simulink model "Full_RC_2"  (Simulink 8.3)
settings: Solver=ode45  StartTime=0.0  StopTime=300000.0  RelTol=1e-3
settings Model: Creator=user  LastModifiedBy=user
settings DataIOCC: SignalLoggingSaveFormat=Dataset
settings DebuggingCC: UnderspecifiedInitializationDetection=Simplified  StateNameClashWarn=none
settings GRTTargetCC: CombineOutputUpdateFcns=on  GRTInterface=off

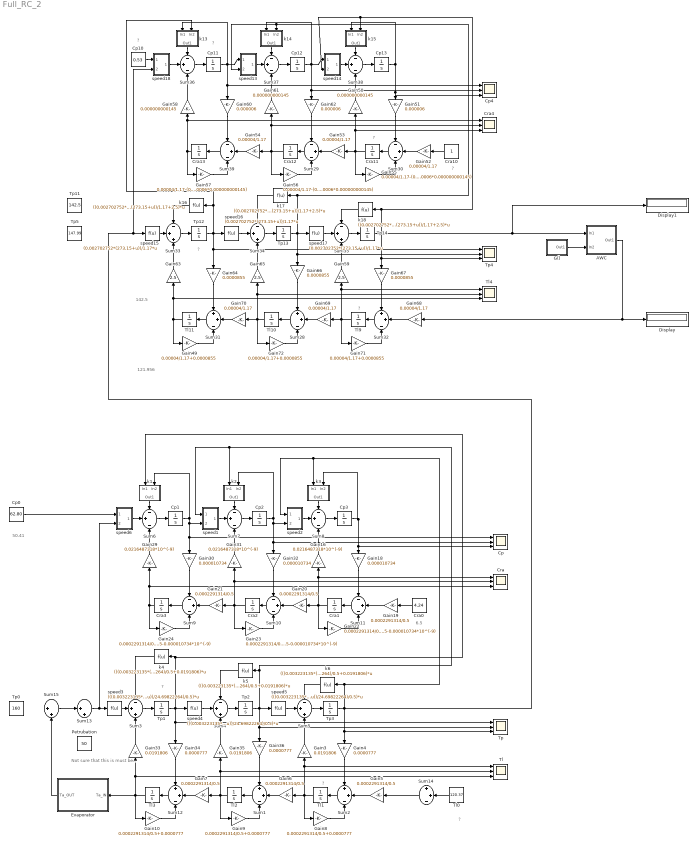
== system Full_RC_2 ==
  note: ?
  note: ?
  note: ?
  note: ?
  note: ?
  note: ?
  note: ?
  note: ?
  note: ?
  note: 50.41
  note: 6.5
  note: 142.5
  note: 121.956
  note: Not sure that
      | this is must be..
  AWC : Subsystem
  Cp : Scope  NumInputPorts=3
      settings: TimeRange=12  YMin=61.5~77~95.34999999999999  YMax=62.5~82~95.37000000000001  SaveName=Cp  DataFormat=Structure
  Cp0 : Constant  Value=62.80
  Cp1 : Integrator  InitialCondition=62.80
  Cp10 : Constant  Value=0.53
  Cp11 : Integrator  InitialCondition=0.665
  Cp12 : Integrator  InitialCondition=0.803
  Cp13 : Integrator  InitialCondition=0.986
  Cp2 : Integrator  InitialCondition=77.79
  Cp3 : Integrator  InitialCondition=96.56
  Cp4 : Scope  NumInputPorts=3
      settings: TimeRange=12  YMin=61.5~77~95.34999999999999  YMax=62.5~82~95.37000000000001  SaveName=Cp1  DataFormat=Structure
  Cra : Scope  NumInputPorts=3
      settings: YMin=4.17~2.4~0.84  YMax=4.28~2.5~1  SaveName=Cra
  Cra0 : Constant  Value=4.24
  Cra1 : Integrator  InitialCondition=4.24
  Cra10 : Constant
  Cra11 : Integrator  InitialCondition=0.827
  Cra12 : Integrator  InitialCondition=0.6862
  Cra13 : Integrator  InitialCondition=0.5696
  Cra2 : Integrator  InitialCondition=2.42
  Cra3 : Integrator  InitialCondition=0.95
  Cra4 : Scope  NumInputPorts=3
      settings: YMin=4.17~2.4~0.84  YMax=4.28~2.5~1  SaveName=Cra1
  Display : Display
  Display1 : Display
  Evaporator : Subsystem
  G() : Subsystem
  Gain10 : Gain  Gain=0.0002291314/0.5+0.0000777
  Gain16 : Gain  Gain=0.0216487318*10^(-9)
  Gain18 : Gain  Gain=0.000010734
  Gain{5..7,19..21} (6 alike) : Gain  Gain=0.0002291314/0.5
  Gain22 : Gain  Gain=0.0002291314/0.5-0.000010734*10^(-9)
  Gain23 : Gain  Gain=0.0002291314/0.5-0.000010734*10^(-9)
  Gain24 : Gain  Gain=0.0002291314/0.5-0.000010734*10^(-9)
  Gain29 : Gain  Gain=0.0216487318*10^(-9)
  Gain3 : Gain  Gain=0.0191806
  Gain30 : Gain  Gain=0.000010734
  Gain31 : Gain  Gain=0.0216487318*10^(-9)
  Gain32 : Gain  Gain=0.000010734
  Gain33 : Gain  Gain=0.0191806
  Gain34 : Gain  Gain=0.0000777
  Gain35 : Gain  Gain=0.0191806
  Gain36 : Gain  Gain=0.0000777
  Gain4 : Gain  Gain=0.0000777
  Gain49 : Gain  Gain=0.00004/1.17+0.0000855
  Gain50 : Gain  Gain=0.000000000145
  Gain51 : Gain  Gain=0.000006
  Gain{52..54,68..70} (6 alike) : Gain  Gain=0.00004/1.17
  Gain55 : Gain  Gain=0.00004/1.17-(0.000006*0.000000000145)
  Gain56 : Gain  Gain=0.00004/1.17-(0.000006*0.000000000145)
  Gain57 : Gain  Gain=0.00004/1.17-(0.000006*0.000000000145)
  Gain58 : Gain  Gain=0.000000000145
  Gain59 : Gain  Gain=2.5
  Gain60 : Gain  Gain=0.000006
  Gain61 : Gain  Gain=0.000000000145
  Gain62 : Gain  Gain=0.000006
  Gain63 : Gain  Gain=2.5
  Gain64 : Gain  Gain=0.0000855
  Gain65 : Gain  Gain=2.5
  Gain66 : Gain  Gain=0.0000855
  Gain67 : Gain  Gain=0.0000855
  Gain71 : Gain  Gain=0.00004/1.17+0.0000855
  Gain72 : Gain  Gain=0.00004/1.17+0.0000855
  Gain8 : Gain  Gain=0.0002291314/0.5+0.0000777
  Gain9 : Gain  Gain=0.0002291314/0.5+0.0000777
  Petrubation : Constant  Value=50
  Sum{1..2,12,14,28,31..32} (7 alike) : Sum  Inputs=++-
  Sum{6..11,29..30,36..39} (12 alike) : Sum  Inputs=-+-
  Sum13 : Sum  Inputs=|++
  Sum15 : Sum  Inputs=|++
  Sum{3..5,33..35} (6 alike) : Sum  Inputs=-++
  Tl : Scope  NumInputPorts=3
      settings: YMin=13~10~8.800000000000001  YMax=15.2~21~10.55  SaveName=Tl
  Tl0 : Constant  Value=120.37
  Tl1 : Integrator  InitialCondition=120.37
  Tl10 : Integrator  InitialCondition=86.23
  Tl11 : Integrator  InitialCondition=111.75
  Tl2 : Integrator  InitialCondition=124.37
  Tl3 : Integrator  InitialCondition=128.38
  Tl4 : Scope  NumInputPorts=3
      settings: YMin=13~10~8.800000000000001  YMax=15.2~21~10.55  SaveName=Tl1
  Tl9 : Integrator  InitialCondition=58.28
  Tp : Scope  NumInputPorts=3
      settings: TimeRange=12  YMin=155.5~145~146  YMax=158.5~152~154.5  SaveName=Tp
  Tp0 : Constant  Value=160
  Tp1 : Integrator  InitialCondition=160
  Tp11 : Constant  Value=142.5
  Tp12 : Integrator  InitialCondition=121.956
  Tp13 : Integrator  InitialCondition=97.4
  Tp14 : Integrator  InitialCondition=69.6  IgnoreLimit=on
  Tp2 : Integrator  InitialCondition=157.34
  Tp3 : Integrator  InitialCondition=153.75  IgnoreLimit=on
  Tp4 : Scope  NumInputPorts=3
      settings: TimeRange=12  YMin=123.005~98.3982~69.9473  YMax=135.953~108.756~77.3101  SaveName=Tp1
  Tp5 : Constant  Value=147.99
  k1 : Subsystem
  k13 : Subsystem
  k14 : Subsystem
  k15 : Subsystem
  k16 : Fcn  Expr=((0.002702752*(273.15+u))/1.17+2.5)*u
  k17 : Fcn  Expr=((0.002702752*(273.15+u))/1.17+2.5)*u
  k18 : Fcn  Expr=((0.002702752*(273.15+u))/1.17+2.5)*u
  k2 : Subsystem
  k3 : Subsystem
  k4 : Fcn  Expr=(((0.003223135*(273+u))/24.69822264)/0.5+0.0191806)*u
  k5 : Fcn  Expr=(((0.003223135*(273+u))/24.69822264)/0.5+0.0191806)*u
  k6 : Fcn  Expr=(((0.003223135*(273+u))/24.69822264)/0.5+0.0191806)*u
  speed1 : Subsystem
  speed13 : Subsystem
  speed14 : Subsystem
  speed15 : Fcn  Expr=(0.002702752*(273.15+u))/1.17*u
  speed16 : Fcn  Expr=(0.002702752*(273.15+u))/1.17*u
  speed17 : Fcn  Expr=(0.002702752*(273.15+u))/1.17*u
  speed18 : Subsystem
  speed2 : Subsystem
  speed3 : Fcn  Expr=(((0.003223135*(273+u))/24.69822264)/0.5)*u
  speed4 : Fcn  Expr=(((0.003223135*(273+u))/24.69822264)/0.5)*u
  speed5 : Fcn  Expr=(((0.003223135*(273+u))/24.69822264)/0.5)*u
  speed6 : Subsystem
  wires:
  Sum6/1 -> Cp1/1
  speed1/1(Out1) -> Sum7/2
  Sum7/1 -> Cp2/1
  speed2/1(Out1) -> Sum8/2
  Sum8/1 -> Cp3/1
  Cp1/1 -> speed1/2(In2), Gain30/1, Cp/1, k1/2(In2)
  Cp2/1 -> speed2/2(In2), Gain32/1, Cp/2, k2/2(In2)
  Gain29/1 -> Sum6/3
  Cp3/1 -> k3/2(In2), Gain18/1, Cp/3
  Gain31/1 -> Sum7/3
  Gain16/1 -> Sum8/3
  Gain30/1 -> Sum9/1
  Gain32/1 -> Sum10/1
  Gain18/1 -> Sum11/1
  Gain19/1 -> Sum11/2
  Sum11/1 -> Cra1/1
  Cra1/1 -> Gain22/1, Gain20/1, Gain16/1, Cra/1
  Gain20/1 -> Sum10/2
  Sum10/1 -> Cra2/1
  Cra2/1 -> Gain23/1, Gain21/1, Gain31/1, Cra/2
  Gain21/1 -> Sum9/2
  Sum9/1 -> Cra3/1
  Cra3/1 -> Gain24/1, Gain29/1, Cra/3
  Gain22/1 -> Sum11/3
  Gain23/1 -> Sum10/3
  Gain24/1 -> Sum9/3
  speed3/1 -> Sum3/2
  k4/1 -> Sum3/1
  Sum3/1 -> Tp1/1
  speed4/1 -> Sum4/2
  k5/1 -> Sum4/1
  Sum4/1 -> Tp2/1
  speed5/1 -> Sum5/2
  k6/1 -> Sum5/1
  Sum5/1 -> Tp3/1
  Gain33/1 -> Sum3/3
  Tp3/1 -> Gain4/1, Tp/3, speed18/2(In2), speed15/1, k6/1, k3/1(In1), speed2/1(In1)
  Gain35/1 -> Sum4/3
  Gain3/1 -> Sum5/3
  Gain34/1 -> Sum12/1
  Gain36/1 -> Sum1/1
  Gain4/1 -> Sum2/1
  Gain5/1 -> Sum2/2
  Sum2/1 -> Tl1/1
  Tl1/1 -> Gain8/1, Gain6/1, Gain3/1, Tl/1
  Gain6/1 -> Sum1/2
  Sum1/1 -> Tl2/1
  Tl2/1 -> Gain9/1, Gain7/1, Gain35/1, Tl/2
  Gain7/1 -> Sum12/2
  Sum12/1 -> Tl3/1
  Tl3/1 -> Evaporator/1(Ta_IN), Gain10/1, Gain33/1, Tl/3
  Gain8/1 -> Sum2/3
  Gain9/1 -> Sum1/3
  Gain10/1 -> Sum12/3
  speed6/1(Out1) -> Sum6/2
  Cp0/1 -> speed6/1(In1)
  k1/1(Out1) -> Sum6/1
  k2/1(Out1) -> Sum7/1
  k3/1(Out1) -> Sum8/1
  Cra0/1 -> Gain19/1
  Sum13/1 -> speed6/2(In2), speed3/1
  G()/1(Out1) -> AWC/2(In2)
  Sum14/1 -> Gain5/1
  Sum15/1 -> Sum13/1
  Tl0/1 -> Sum14/2
  Tp2/1 -> Gain36/1, Tp/2, k5/1, speed1/1(In1), k2/1(In1), speed5/1
  Tp1/1 -> Gain34/1, Tp/1, k4/1, k1/1(In1), speed4/1
  Evaporator/1(Ta_OUT) -> Sum15/2
  Sum36/1 -> Cp11/1
  speed13/1(Out1) -> Sum37/2
  Sum37/1 -> Cp12/1
  speed14/1(Out1) -> Sum38/2
  Sum38/1 -> Cp13/1
  Cp11/1 -> Cp4/1, Gain60/1, speed13/1(In1), k13/1(In1)
  Cp12/1 -> Cp4/2, Gain62/1, speed14/1(In1), k14/1(In1)
  Gain58/1 -> Sum36/3
  Cp13/1 -> Cp4/3, Gain51/1, k15/1(In1)
  Gain61/1 -> Sum37/3
  Gain50/1 -> Sum38/3
  Gain60/1 -> Sum39/1
  Gain62/1 -> Sum29/1
  Gain51/1 -> Sum30/1
  Gain52/1 -> Sum30/2
  Sum30/1 -> Cra11/1
  Cra11/1 -> Gain55/1, Gain53/1, Cra4/3, Gain50/1
  Gain53/1 -> Sum29/2
  Sum29/1 -> Cra12/1
  Cra12/1 -> Gain56/1, Gain54/1, Cra4/2, Gain61/1
  Gain54/1 -> Sum39/2
  Sum39/1 -> Cra13/1
  Cra13/1 -> Gain57/1, Cra4/1, Gain58/1
  Gain55/1 -> Sum30/3
  Gain56/1 -> Sum29/3
  Gain57/1 -> Sum39/3
  speed15/1 -> Sum33/2
  k16/1 -> Sum33/1
  Sum33/1 -> Tp12/1
  speed16/1 -> Sum34/2
  k17/1 -> Sum34/1
  Sum34/1 -> Tp13/1
  speed17/1 -> Sum35/2
  k18/1 -> Sum35/1
  Sum35/1 -> Tp14/1
  Tp12/1 -> Gain64/1, Tp4/1, k16/1, k13/2(In2), speed16/1
  Tp13/1 -> Gain66/1, Tp4/2, k17/1, speed13/2(In2), k14/2(In2), speed17/1
  Gain63/1 -> Sum33/3
  Gain65/1 -> Sum34/3
  Gain59/1 -> Sum35/3
  Gain64/1 -> Sum31/1
  Gain66/1 -> Sum28/1
  Gain67/1 -> Sum32/1
  Gain68/1 -> Sum32/2
  Sum32/1 -> Tl9/1
  Tl9/1 -> Gain71/1, Gain69/1, Tl4/1, Gain59/1
  Gain69/1 -> Sum28/2
  Sum28/1 -> Tl10/1
  Tl10/1 -> Gain72/1, Gain70/1, Tl4/2, Gain65/1
  Gain70/1 -> Sum31/2
  Sum31/1 -> Tl11/1
  Tl11/1 -> Gain49/1, Gain63/1, Tl4/3
  Gain71/1 -> Sum32/3
  Gain72/1 -> Sum28/3
  Gain49/1 -> Sum31/3
  speed18/1(Out1) -> Sum36/2
  Cp10/1 -> speed18/1(In1)
  k13/1(Out1) -> Sum36/1
  k14/1(Out1) -> Sum37/1
  k15/1(Out1) -> Sum38/1
  Cra10/1 -> Gain52/1
  Tp14/1 -> AWC/1(In1), Display1/1, Gain67/1, Tp4/3, k18/1, k15/2(In2), speed14/2(In2)
  AWC/1(Out1) -> Display/1, Gain68/1

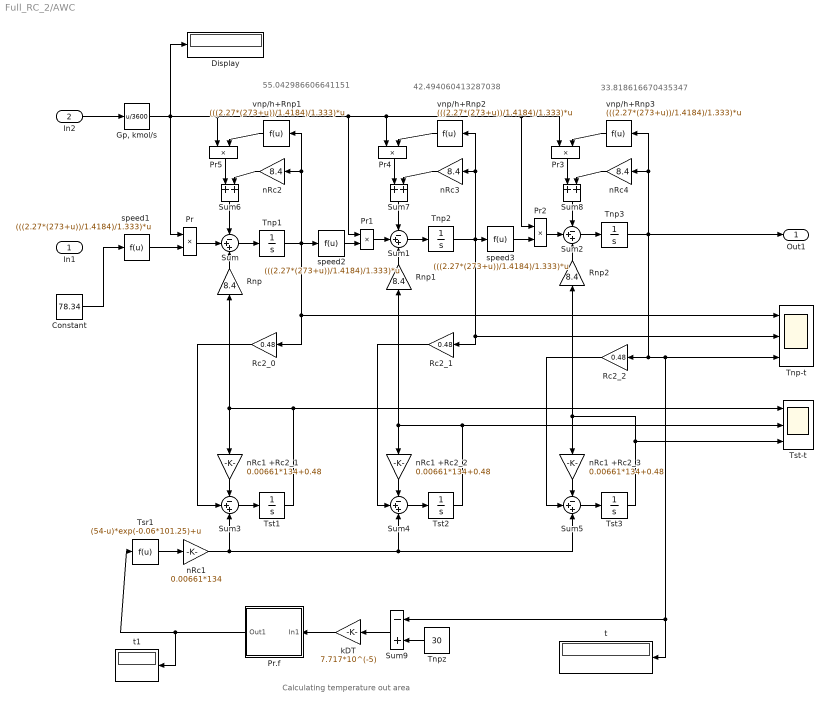
== system Full_RC_2/AWC ==
  note: 33.818616670435347
  note: 42.494060413287038
  note: 55.042986606641151
  note: Calculating temperature out area
  In1 : Inport
  In2 : Inport  Port=2
  Constant : Constant  Value=78.34
  Display : Display
  "Gp, kmol/s" : Fcn  Expr=u/3600
  Pr{,1..5} (6 alike) : Product  RndMeth=Zero
  Pr.f : Subsystem
  Rc2_0 : Gain  Gain=0.48
  Rc2_1 : Gain  Gain=0.48
  Rc2_2 : Gain  Gain=0.48
  Rnp : Gain  Gain=8.4
  Rnp1 : Gain  Gain=8.4
  Rnp2 : Gain  Gain=8.4
  Sum{,1..5} (6 alike) : Sum  Inputs=-++
  Sum6 : Sum
  Sum7 : Sum
  Sum8 : Sum
  Sum9 : Sum  Inputs=-+
  Tnp-t : Scope  NumInputPorts=3
      settings: YMin=52.458~37.745~29.975  YMax=52.466~37.7725~30.025  SaveName=ScopeData8
  Tnp1 : Integrator  InitialCondition=55.042986606641151
  Tnp2 : Integrator  InitialCondition=42.494060413287038
  Tnp3 : Integrator  InitialCondition=33.818616670435347
  Tnpz : Constant  Value=30
  Tsr1 : Fcn  Expr=(54-u)*exp(-0.06*101.25)+u
  Tst-t : Scope  NumInputPorts=3
      settings: YMin=320.767~573.618~826.668  YMax=354.532~633.998~913.686  SaveName=ScopeData9
  Tst1 : Integrator  InitialCondition=30.749212884999000
  Tst2 : Integrator  InitialCondition=26.338794670104530
  Tst3 : Integrator  InitialCondition=23.289742144317184
  kDT : Gain  Gain=7.717*10^(-5)
  nRc1 : Gain  Gain=0.00661*134
  nRc1 +Rc2_1 : Gain  Gain=0.00661*134+0.48
  nRc1 +Rc2_2 : Gain  Gain=0.00661*134+0.48
  nRc1 +Rc2_3 : Gain  Gain=0.00661*134+0.48
  nRc2 : Gain  Gain=8.4
  nRc3 : Gain  Gain=8.4
  nRc4 : Gain  Gain=8.4
  speed1 : Fcn  Expr=(((2.27*(273+u))/1.4184)/1.333)*u
  speed2 : Fcn  Expr=(((2.27*(273+u))/1.4184)/1.333)*u
  speed3 : Fcn  Expr=(((2.27*(273+u))/1.4184)/1.333)*u
  t : Display
  t1 : Display
  vnp/h+Rnp1 : Fcn  Expr=(((2.27*(273+u))/1.4184)/1.333)*u
  vnp/h+Rnp2 : Fcn  Expr=(((2.27*(273+u))/1.4184)/1.333)*u
  vnp/h+Rnp3 : Fcn  Expr=(((2.27*(273+u))/1.4184)/1.333)*u
  Out1 : Outport
  wires:
  Sum/1 -> Tnp1/1
  Tnp1/1 -> speed2/1, Rc2_0/1, Tnp-t/1, vnp/h+Rnp1/1, nRc2/1
  Sum1/1 -> Tnp2/1
  Tnp2/1 -> speed3/1, Rc2_1/1, Tnp-t/2, vnp/h+Rnp2/1, nRc3/1
  Sum2/1 -> Tnp3/1
  Tnp3/1 -> vnp/h+Rnp3/1, nRc4/1, Out1/1, Rc2_2/1, Tnp-t/3, t/1, Sum9/1
  Rnp1/1 -> Sum1/3
  Rnp2/1 -> Sum2/3
  nRc1 +Rc2_1/1 -> Sum3/1
  Sum3/1 -> Tst1/1
  nRc1 +Rc2_2/1 -> Sum4/1
  Sum4/1 -> Tst2/1
  Tst2/1 -> Rnp1/1, nRc1 +Rc2_2/1, Tst-t/2
  nRc1 +Rc2_3/1 -> Sum5/1
  Sum5/1 -> Tst3/1
  nRc1/1 -> Sum3/3, Sum4/3, Sum5/3
  Rnp/1 -> Sum/3
  Tst1/1 -> nRc1 +Rc2_1/1, Rnp/1, Tst-t/1
  Tst3/1 -> Rnp2/1, nRc1 +Rc2_3/1, Tst-t/3
  Rc2_1/1 -> Sum4/2
  Rc2_2/1 -> Sum5/2
  Rc2_0/1 -> Sum3/2
  speed1/1 -> Pr/2
  "Gp, kmol/s"/1 -> Display/1, Pr/1, Pr5/1, Pr2/1, Pr3/1, Pr4/1, Pr1/1
  Pr/1 -> Sum/2
  Pr1/1 -> Sum1/2
  speed2/1 -> Pr1/2
  Pr2/1 -> Sum2/2
  speed3/1 -> Pr2/2
  vnp/h+Rnp3/1 -> Pr3/2
  vnp/h+Rnp2/1 -> Pr4/2
  vnp/h+Rnp1/1 -> Pr5/2
  Pr5/1 -> Sum6/1
  Sum6/1 -> Sum/1
  nRc2/1 -> Sum6/2
  nRc3/1 -> Sum7/2
  Pr4/1 -> Sum7/1
  Sum7/1 -> Sum1/1
  nRc4/1 -> Sum8/2
  Pr3/1 -> Sum8/1
  Sum8/1 -> Sum2/1
  Sum9/1 -> kDT/1
  Tnpz/1 -> Sum9/2
  Pr.f/1(Out1) -> t1/1, Tsr1/1
  kDT/1 -> Pr.f/1(In1)
  Tsr1/1 -> nRc1/1
  In2/1 -> "Gp, kmol/s"/1
  Constant/1 -> speed1/1

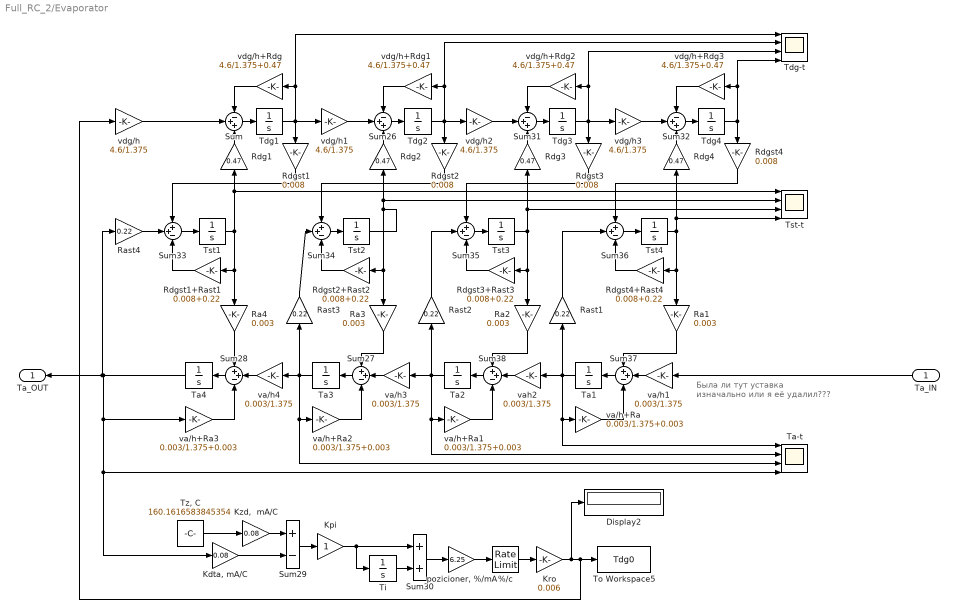
== system Full_RC_2/Evaporator ==
  note: Была ли тут уставка изначально или я её удалил???
  Ta_IN : Inport
  %/c : RateLimiter  RisingSlewLimit=5  FallingSlewLimit=-5  SampleTimeMode=inherited
  Display2 : Display
  "Kdta, mA/C" : Gain  Gain=0.08
  Kpi : Gain
  Kro : Gain  Gain=0.006
  "Kzd,  mA/C" : Gain  Gain=0.08
  Ra{1..4} (4 alike) : Gain  Gain=0.003
  Rast{1..4} (4 alike) : Gain  Gain=0.22
  Rdg{1..4} (4 alike) : Gain  Gain=0.47
  Rdgst{1..4} (4 alike) : Gain  Gain=0.008
  Rdgst1+Rast1 : Gain  Gain=0.008+0.22
  Rdgst2+Rast2 : Gain  Gain=0.008+0.22
  Rdgst3+Rast3 : Gain  Gain=0.008+0.22
  Rdgst4+Rast4 : Gain  Gain=0.008+0.22
  Sum{,26,31..32} (4 alike) : Sum  Inputs=-++
  Sum{27..28,33..38} (8 alike) : Sum  Inputs=++-
  Sum29 : Sum  Inputs=+-
  Sum30 : Sum
  Ta-t : Scope  NumInputPorts=4
      settings: YMin=-5~-5~100~100  YMax=5~5~165~165  SaveName=ScopeData11
  Ta1 : Integrator  InitialCondition=136.285
  Ta2 : Integrator  InitialCondition=144.19
  Ta3 : Integrator  InitialCondition=152.09
  Ta4 : Integrator  InitialCondition=160
  Tdg-t : Scope  NumInputPorts=4
      settings: YMin=-5~-5~-5~-5  YMax=5~5~5~5  SaveName=ScopeData12
  Tdg1 : Integrator  InitialCondition=283.3065209436467
  Tdg2 : Integrator  InitialCondition=267.8966165589237
  Tdg3 : Integrator  InitialCondition=253.6715917846216
  Tdg4 : Integrator  InitialCondition=240.5403403000344
  Ti : Integrator  InitialCondition=8000  UpperSaturationLimit=8012  LowerSaturationLimit=6012
  To Workspace5 : ToWorkspace  VariableName=Tdg0  SampleTime=-1
  Tst-t : Scope  NumInputPorts=4
      settings: YMin=-5~-5~-5~-5  YMax=5~5~5~5  SaveName=ScopeData13
  Tst1 : Integrator  InitialCondition=164.4825307550351
  Tst2 : Integrator  InitialCondition=158.2090959868120
  Tst3 : Integrator  InitialCondition=152.4180305285302
  Tst4 : Integrator  InitialCondition=147.0722446263660
  "Tz, C" : Constant  Value=160.1616583845354
  "pozicioner, %/mA" : Gain  Gain=6.25
  va/h+Ra{,1..3} (4 alike) : Gain  Gain=0.003/1.375+0.003
  va/h1 : Gain  Gain=0.003/1.375
  va/h3 : Gain  Gain=0.003/1.375
  va/h4 : Gain  Gain=0.003/1.375
  vah2 : Gain  Gain=0.003/1.375
  vdg/h{,1..3} (4 alike) : Gain  Gain=4.6/1.375
  vdg/h+Rdg{,1..3} (4 alike) : Gain  Gain=4.6/1.375+0.47
  Ta_OUT : Outport
  wires:
  Sum/1 -> Tdg1/1
  vdg/h2/1 -> Sum31/2
  Sum32/1 -> Tdg4/1
  Tdg2/1 -> vdg/h+Rdg1/1, Tdg-t/2, Rdgst2/1, vdg/h2/1
  Sum26/1 -> Tdg2/1
  vdg/h3/1 -> Sum32/2
  vdg/h/1 -> Sum/2
  Tdg1/1 -> vdg/h+Rdg/1, Tdg-t/1, vdg/h1/1, Rdgst1/1
  vdg/h+Rdg2/1 -> Sum31/1
  vdg/h+Rdg3/1 -> Sum32/1
  Tdg4/1 -> vdg/h+Rdg3/1, Tdg-t/4, Rdgst4/1
  Rdg1/1 -> Sum/3
  Rdg2/1 -> Sum26/3
  Rdg3/1 -> Sum31/3
  Rdg4/1 -> Sum32/3
  vdg/h+Rdg1/1 -> Sum26/1
  Sum33/1 -> Tst1/1
  Sum34/1 -> Tst2/1
  Tdg3/1 -> vdg/h+Rdg2/1, Tdg-t/3, vdg/h3/1, Rdgst3/1
  vdg/h1/1 -> Sum26/2
  Sum35/1 -> Tst3/1
  vdg/h+Rdg/1 -> Sum/1
  Sum31/1 -> Tdg3/1
  Rdgst3+Rast3/1 -> Sum35/3
  Tst1/1 -> Rdgst1+Rast1/1, Ra4/1, Rdg1/1, Tst-t/1
  Rdgst1+Rast1/1 -> Sum33/3
  Tst3/1 -> Rdgst3+Rast3/1, Ra2/1, Rdg3/1, Tst-t/3
  Tst2/1 -> Rdg2/1, Tst-t/2, Rdgst2+Rast2/1, Ra3/1
  Rdgst1/1 -> Sum33/1
  Rdgst2/1 -> Sum34/1
  Tst4/1 -> Rdgst4+Rast4/1, Ra1/1, Rdg4/1, Tst-t/4
  Rdgst4/1 -> Sum36/1
  Rdgst2+Rast2/1 -> Sum34/3
  va/h1/1 -> Sum37/2
  va/h+Ra/1 -> Sum37/3
  Rdgst3/1 -> Sum35/1
  Sum36/1 -> Tst4/1
  Rdgst4+Rast4/1 -> Sum36/3
  Ti/1 -> Sum30/2
  Ta4/1 -> Ta_OUT/1, Rast4/1, va/h+Ra3/1, Ta-t/4, "Kdta, mA/C"/1
  Rast1/1 -> Sum36/2
  Ra2/1 -> Sum38/1
  Ta2/1 -> va/h+Ra1/1, Ta-t/2, va/h3/1, Rast2/1
  va/h+Ra3/1 -> Sum28/3
  Ta1/1 -> Ta-t/1, va/h+Ra/1, Rast1/1, vah2/1
  va/h+Ra2/1 -> Sum27/3
  Rast3/1 -> Sum34/2
  Sum38/1 -> Ta2/1
  va/h4/1 -> Sum28/2
  Sum37/1 -> Ta1/1
  va/h3/1 -> Sum27/2
  Ta3/1 -> va/h+Ra2/1, Ta-t/3, va/h4/1, Rast3/1
  Rast2/1 -> Sum35/2
  "Tz, C"/1 -> "Kzd,  mA/C"/1
  "Kdta, mA/C"/1 -> Sum29/2
  %/c/1 -> Kro/1
  Ta_IN/1 -> va/h1/1
  "Kzd,  mA/C"/1 -> Sum29/1
  Sum28/1 -> Ta4/1
  Rast4/1 -> Sum33/2
  Sum27/1 -> Ta3/1
  va/h+Ra1/1 -> Sum38/3
  "pozicioner, %/mA"/1 -> %/c/1
  Ra3/1 -> Sum27/1
  Sum29/1 -> Kpi/1
  Kpi/1 -> Sum30/1, Ti/1
  Ra4/1 -> Sum28/1
  Sum30/1 -> "pozicioner, %/mA"/1
  Kro/1 -> To Workspace5/1, vdg/h/1, Display2/1
  Ra1/1 -> Sum37/1
  vah2/1 -> Sum38/2

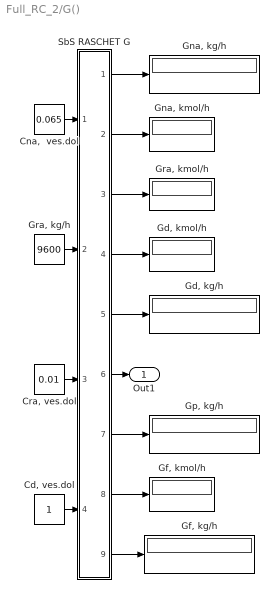
== system Full_RC_2/G() ==
  "Cd, ves.dol" : Constant
  "Cna,  ves.dol" : Constant  Value=0.065
  "Cra, ves.dol" : Constant  Value=0.01
  "Gd, kg/h" : Display
  "Gd, kmol/h" : Display
  "Gf, kg/h" : Display
  "Gf, kmol/h" : Display
  "Gna, kg/h" : Display
  "Gna, kmol/h" : Display
  "Gp, kg/h" : Display
  "Gra, kg/h" : Constant  Value=9600
  "Gra, kmol/h" : Display
  SbS RASCHET G : Subsystem
  Out1 : Outport
  wires:
  SbS RASCHET G/2(Out2) -> "Gna, kmol/h"/1
  "Cra, ves.dol"/1 -> SbS RASCHET G/3(In3)
  "Cna,  ves.dol"/1 -> SbS RASCHET G/1(In1)
  SbS RASCHET G/1(Out1) -> "Gna, kg/h"/1
  "Cd, ves.dol"/1 -> SbS RASCHET G/4(In4)
  "Gra, kg/h"/1 -> SbS RASCHET G/2(In2)
  SbS RASCHET G/7(Out7) -> "Gp, kg/h"/1
  SbS RASCHET G/9(Out9) -> "Gf, kg/h"/1
  SbS RASCHET G/8(Out8) -> "Gf, kmol/h"/1
  SbS RASCHET G/4(Out4) -> "Gd, kmol/h"/1
  SbS RASCHET G/5(Out5) -> "Gd, kg/h"/1
  SbS RASCHET G/3(Out3) -> "Gra, kmol/h"/1
  SbS RASCHET G/6(Out6) -> Out1/1

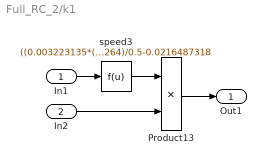
== system Full_RC_2/k1 ==
  In1 : Inport
  In2 : Inport  Port=2
  Product13 : Product  SaturateOnIntegerOverflow=on  InputSameDT=on  OutDataTypeStr=Inherit: Same as first input
  speed3 : Fcn  Expr=((0.003223135*(273+u))/24.69822264)/0.5-0.0216487318
  Out1 : Outport
  wires:
  Product13/1 -> Out1/1
  speed3/1 -> Product13/1
  In1/1 -> speed3/1
  In2/1 -> Product13/2

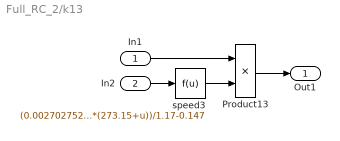
== system Full_RC_2/k13 ==
  In1 : Inport
  In2 : Inport  Port=2
  Product13 : Product  SaturateOnIntegerOverflow=on  InputSameDT=on  OutDataTypeStr=Inherit: Same as first input
  speed3 : Fcn  Expr=(0.002702752*(273.15+u))/1.17-0.147
  Out1 : Outport
  wires:
  Product13/1 -> Out1/1
  speed3/1 -> Product13/2
  In2/1 -> speed3/1
  In1/1 -> Product13/1

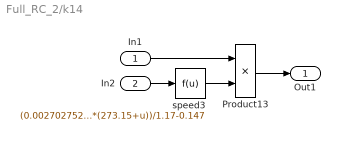
== system Full_RC_2/k14 ==
  In1 : Inport
  In2 : Inport  Port=2
  Product13 : Product  SaturateOnIntegerOverflow=on  InputSameDT=on  OutDataTypeStr=Inherit: Same as first input
  speed3 : Fcn  Expr=(0.002702752*(273.15+u))/1.17-0.147
  Out1 : Outport
  wires:
  In1/1 -> Product13/1
  In2/1 -> speed3/1
  speed3/1 -> Product13/2
  Product13/1 -> Out1/1

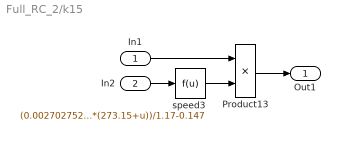
== system Full_RC_2/k15 ==
  In1 : Inport
  In2 : Inport  Port=2
  Product13 : Product  SaturateOnIntegerOverflow=on  InputSameDT=on  OutDataTypeStr=Inherit: Same as first input
  speed3 : Fcn  Expr=(0.002702752*(273.15+u))/1.17-0.147
  Out1 : Outport
  wires:
  Product13/1 -> Out1/1
  speed3/1 -> Product13/2
  In2/1 -> speed3/1
  In1/1 -> Product13/1

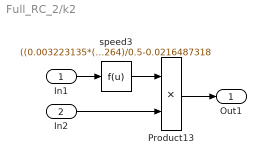
== system Full_RC_2/k2 ==
  In1 : Inport
  In2 : Inport  Port=2
  Product13 : Product  SaturateOnIntegerOverflow=on  InputSameDT=on  OutDataTypeStr=Inherit: Same as first input
  speed3 : Fcn  Expr=((0.003223135*(273+u))/24.69822264)/0.5-0.0216487318
  Out1 : Outport
  wires:
  Product13/1 -> Out1/1
  speed3/1 -> Product13/1
  In1/1 -> speed3/1
  In2/1 -> Product13/2

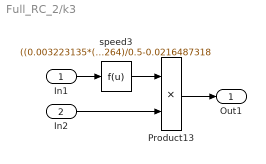
== system Full_RC_2/k3 ==
  In1 : Inport
  In2 : Inport  Port=2
  Product13 : Product  SaturateOnIntegerOverflow=on  InputSameDT=on  OutDataTypeStr=Inherit: Same as first input
  speed3 : Fcn  Expr=((0.003223135*(273+u))/24.69822264)/0.5-0.0216487318
  Out1 : Outport
  wires:
  Product13/1 -> Out1/1
  speed3/1 -> Product13/1
  In1/1 -> speed3/1
  In2/1 -> Product13/2

== system Full_RC_2/speed1 ==
  In1 : Inport
  In2 : Inport  Port=2
  Product13 : Product  SaturateOnIntegerOverflow=on  InputSameDT=on  OutDataTypeStr=Inherit: Same as first input
  speed3 : Fcn  Expr=((0.003223135*(273+u))/24.69822264)/0.5
  Out1 : Outport
  wires:
  Product13/1 -> Out1/1
  In2/1 -> Product13/2
  speed3/1 -> Product13/1
  In1/1 -> speed3/1

== system Full_RC_2/speed13 ==
  In1 : Inport
  In2 : Inport  Port=2
  Product13 : Product  SaturateOnIntegerOverflow=on  InputSameDT=on  OutDataTypeStr=Inherit: Same as first input
  speed3 : Fcn  Expr=(0.002702752*(273.15+u))/1.17
  Out1 : Outport
  wires:
  Product13/1 -> Out1/1
  speed3/1 -> Product13/2
  In2/1 -> speed3/1
  In1/1 -> Product13/1

== system Full_RC_2/speed14 ==
  In1 : Inport
  In2 : Inport  Port=2
  Product13 : Product  SaturateOnIntegerOverflow=on  InputSameDT=on  OutDataTypeStr=Inherit: Same as first input
  speed3 : Fcn  Expr=(0.002702752*(273.15+u))/1.17
  Out1 : Outport
  wires:
  In1/1 -> Product13/1
  In2/1 -> speed3/1
  speed3/1 -> Product13/2
  Product13/1 -> Out1/1

== system Full_RC_2/speed18 ==
  In1 : Inport
  In2 : Inport  Port=2
  Product13 : Product  SaturateOnIntegerOverflow=on  InputSameDT=on  OutDataTypeStr=Inherit: Same as first input
  speed3 : Fcn  Expr=(0.002702752*(273.15+u))/1.17
  Out1 : Outport
  wires:
  In1/1 -> Product13/1
  In2/1 -> speed3/1
  speed3/1 -> Product13/2
  Product13/1 -> Out1/1

== system Full_RC_2/speed2 ==
  In1 : Inport
  In2 : Inport  Port=2
  Product13 : Product  SaturateOnIntegerOverflow=on  InputSameDT=on  OutDataTypeStr=Inherit: Same as first input
  speed3 : Fcn  Expr=((0.003223135*(273+u))/24.69822264)/0.5
  Out1 : Outport
  wires:
  Product13/1 -> Out1/1
  In2/1 -> Product13/2
  speed3/1 -> Product13/1
  In1/1 -> speed3/1

== system Full_RC_2/speed6 ==
  In1 : Inport
  In2 : Inport  Port=2
  Product13 : Product  SaturateOnIntegerOverflow=on  InputSameDT=on  OutDataTypeStr=Inherit: Same as first input
  speed3 : Fcn  Expr=((0.003223135*(273+u))/24.69822264)/0.5
  Out1 : Outport
  wires:
  In1/1 -> Product13/1
  In2/1 -> speed3/1
  speed3/1 -> Product13/2
  Product13/1 -> Out1/1

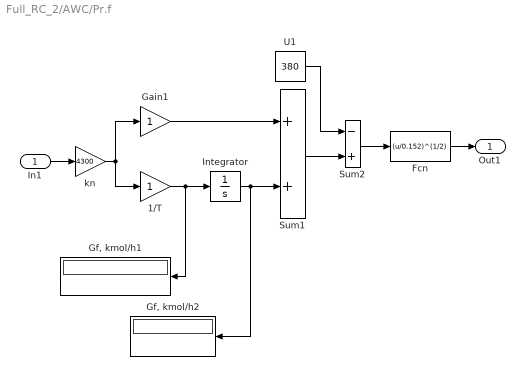
== system Full_RC_2/AWC/Pr.f ==
  In1 : Inport
  1/T : Gain
  Fcn : Fcn  Expr=(u/0.152)^(1/2)
  Gain1 : Gain
  "Gf, kmol/h1" : Display
  "Gf, kmol/h2" : Display
  Integrator : Integrator  InitialCondition=403.6
  Sum1 : Sum
  Sum2 : Sum  Inputs=-+
  U1 : Constant  Value=380
  kn : Gain  Gain=4300
  Out1 : Outport
  wires:
  kn/1 -> 1/T/1, Gain1/1
  1/T/1 -> Integrator/1, "Gf, kmol/h1"/1
  Integrator/1 -> Sum1/2, "Gf, kmol/h2"/1
  Gain1/1 -> Sum1/1
  Sum1/1 -> Sum2/2
  U1/1 -> Sum2/1
  In1/1 -> kn/1
  Fcn/1 -> Out1/1
  Sum2/1 -> Fcn/1

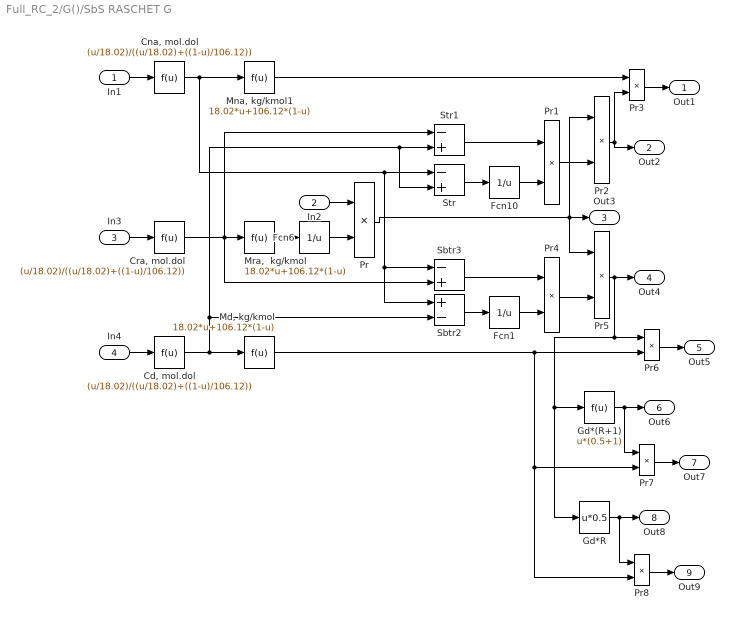
== system Full_RC_2/G()/SbS RASCHET G ==
  In1 : Inport
  In2 : Inport  Port=2
  In3 : Inport  Port=3
  In4 : Inport  Port=4
  "Cd, mol.dol" : Fcn  Expr=(u/18.02)/((u/18.02)+((1-u)/106.12))
  "Cna, mol.dol" : Fcn  Expr=(u/18.02)/((u/18.02)+((1-u)/106.12))
  "Cra, mol.dol" : Fcn  Expr=(u/18.02)/((u/18.02)+((1-u)/106.12))
  Fcn1 : Fcn  Expr=1/u
  Fcn10 : Fcn  Expr=1/u
  Fcn6 : Fcn  Expr=1/u
  Gd*(R+1) : Fcn  Expr=u*(0.5+1)
  Gd*R : Fcn  Expr=u*0.5
  "Md, kg/kmol" : Fcn  Expr=18.02*u+106.12*(1-u)
  "Mna, kg/kmol1" : Fcn  Expr=18.02*u+106.12*(1-u)
  "Mra,  kg/kmol" : Fcn  Expr=18.02*u+106.12*(1-u)
  Pr{,1..8} (9 alike) : Product  RndMeth=Zero
  Sbtr2 : Sum  Inputs=+-
  Sbtr3 : Sum  Inputs=-+
  Str : Sum  Inputs=-+
  Str1 : Sum  Inputs=-+
  Out1 : Outport
  Out2 : Outport  Port=2
  Out3 : Outport  Port=3
  Out4 : Outport  Port=4
  Out5 : Outport  Port=5
  Out6 : Outport  Port=6
  Out7 : Outport  Port=7
  Out8 : Outport  Port=8
  Out9 : Outport  Port=9
  wires:
  "Mna, kg/kmol1"/1 -> Pr3/1
  "Cna, mol.dol"/1 -> "Mna, kg/kmol1"/1, Str/1, Sbtr3/1, Sbtr2/1
  "Cra, mol.dol"/1 -> "Mra,  kg/kmol"/1, Str1/1, Sbtr3/2
  "Cd, mol.dol"/1 -> "Md, kg/kmol"/1, Str1/2, Str/2, Sbtr2/2
  "Mra,  kg/kmol"/1 -> Fcn6/1
  Fcn6/1 -> Pr/2
  Pr/1 -> Pr2/1, Out3/1, Pr5/1
  Str/1 -> Fcn10/1
  Fcn10/1 -> Pr1/2
  Pr2/1 -> Out2/1, Pr3/2
  Pr1/1 -> Pr2/2
  Str1/1 -> Pr1/1
  Fcn1/1 -> Pr4/2
  Pr5/1 -> Pr6/1, Gd*(R+1)/1, Gd*R/1, Out4/1
  Pr4/1 -> Pr5/2
  "Md, kg/kmol"/1 -> Pr6/2, Pr7/2, Pr8/2
  Sbtr2/1 -> Fcn1/1
  Sbtr3/1 -> Pr4/1
  Gd*(R+1)/1 -> Pr7/1, Out6/1
  Gd*R/1 -> Pr8/1, Out8/1
  In1/1 -> "Cna, mol.dol"/1
  Pr3/1 -> Out1/1
  In2/1 -> Pr/1
  In3/1 -> "Cra, mol.dol"/1
  Pr6/1 -> Out5/1
  In4/1 -> "Cd, mol.dol"/1
  Pr7/1 -> Out7/1
  Pr8/1 -> Out9/1
